simulink model "gm_hybrid_lht_vnl"  (R2019b)
settings: Solver=FixedStepDiscrete  StartTime=0.0  StopTime=inf  FixedStep=1/120e6  RelTol=1e-3
undefined symbols (not defined in the file or in its folder): bt, height, nTheta, width
libraries: hdlsllib x327, simulink x213, hdlmdlgenlib x7, dspsrcs4 x1
(part 1 of 14)
settings Model: SimulationMode=accelerator  ExtModeTrigDuration=100  Creator=rgb11127  LastModifiedBy=rgb11127
settings DataIOCC: SaveOutput=off  SaveTime=off  ReturnWorkspaceOutputs=off  StateSaveName=tmp_raccel_xout  SignalLoggingName=tmp_raccel_logsout
settings OptimizationCC: BlockReduction=off  ConditionallyExecuteInputs=off  DefaultParameterBehavior=Inlined  EfficientMapNaN2IntZero=off
settings DebuggingCC: AlgebraicLoopMsg=error  InheritedTsInSrcMsg=none  SingleTaskRateTransMsg=error  ArithmeticOperatorsInVariantConditions=warning
settings HardwareCC: ProdBitPerPointer=32  ProdBitPerSizeT=32  ProdBitPerPtrDiffT=32  ProdLargestAtomicFloat=None  ProdIntDivRoundTo=Undefined  ProdEndianess=Unspecified  ProdWordSize=32  ProdHWDeviceType=ASIC/FPGA->ASIC/FPGA  TargetBitPerPointer=64  TargetBitPerSizeT=64  TargetBitPerPtrDiffT=64  TargetLongLongMode=on  TargetIntDivRoundTo=Zero  TargetEndianess=LittleEndian  TargetWordSize=64  TargetHWDeviceType=Custom Processor->MATLAB Host Computer  ProdEqTarget=off
settings SFSimCC: CustomCodeUndefinedFunction=UseInterfaceOnly
settings RTWCC: SystemTargetFile=raccel.tlc  TemplateMakefile=raccel_default_tmf  RTWVerbose=off  RTWUseSimCustomCode=on
settings CodeAppCC: GenerateComments=off  MaxIdLength=128
settings RaccelTargetCC: GeneratePreprocessorConditionals=Use local settings  MultiInstanceERTCode=off  PreserveStateflowLocalDataDimensions=off  ExtModeMexArgs='', 0, 56287  ENABLE_SLEXEC_SSBRIDGE=1  RTWCAPIParams=on

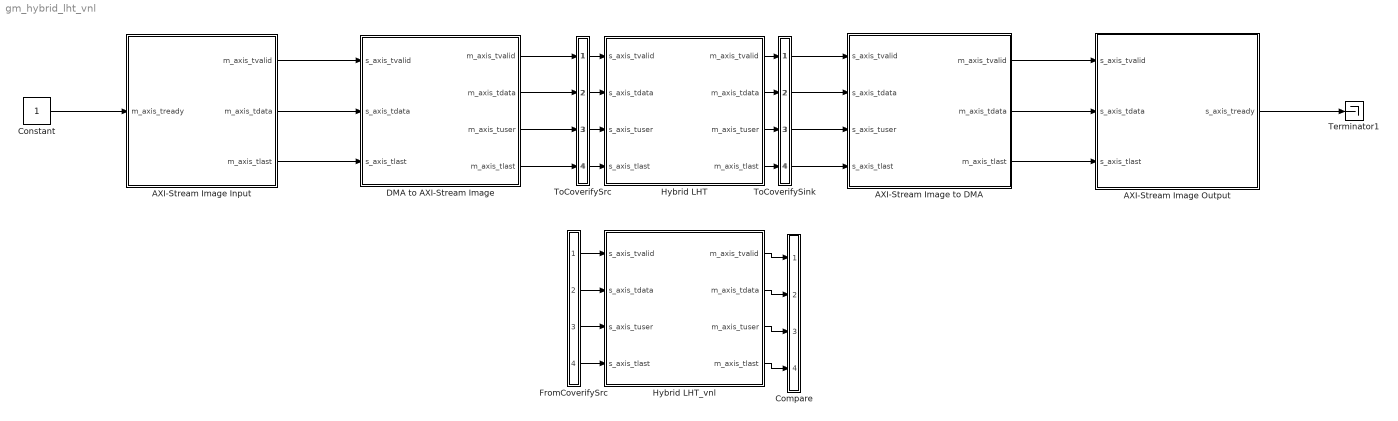
== system gm_hybrid_lht_vnl ==
  AXI-Stream Image Input : Subsystem  mask{image=bt.inputImage, clk=1/120e6}
      mask prompts: image "Input Image:"; clk "Clock Rate:"
      mask init:
      | [height, width] = size(image);
      mask DialogControl DescGroupVar Prompt: AXI-Stream Image Input
      mask DialogControl DescTextVar Prompt: This block simulates an AXI-Stream image input for interfacing to a hardware accelerator or IP Core.
      mask DialogControl ParameterGroupVar Prompt: Main
  AXI-Stream Image Output : Subsystem  mask{height=bt.nRho, width=bt.nTheta, clk=1/120e6, d=0}
      mask prompts: height "Image Height:"; width "Image Width:"; clk "Clock Rate:"; d "Frame Capture Number"
      mask DialogControl DescGroupVar Prompt: AXI-Stream Image Output
      mask DialogControl DescTextVar Prompt: Image output using the AXI-Stream interface. Simulates an AXI DMA write channel.
      mask DialogControl ParameterGroupVar Prompt: Main
  AXI-Stream Image to DMA : Subsystem  mask{height=bt.nRho, width=bt.nTheta}
      mask prompts: height "Image Height"; width "Image Width"
      mask DialogControl DescGroupVar Prompt: AXI-Stream Image to DMA
      mask DialogControl DescTextVar Prompt: Converts from the AXI-Stream video standard to AXI-Stream DMA packet.
      mask DialogControl Container2 Prompt: Main
  Compare : Subsystem
      mask Display: disp('')
  Constant : Constant  OutDataTypeStr=boolean  SampleTime=-1
  DMA to AXI-Stream Image : Subsystem  mask{height=bt.height, width=bt.width}
      mask prompts: height "Image Height:"; width "Image Width:"
      mask DialogControl DescGroupVar Prompt: DMA to AXI-Stream Image
      mask DialogControl DescTextVar Prompt: Converts an DMA AXI-Stream packet to the AXI-Stream video standard.
      mask DialogControl Container2 Prompt: Main
  FromCoverifySrc : Subsystem
      mask Display: disp('')
  Hybrid LHT : Subsystem
  Hybrid LHT_vnl : Subsystem
  Terminator1 : Terminator
  ToCoverifySink : Subsystem
      mask Display: disp('')
  ToCoverifySrc : Subsystem
      mask Display: disp('')
  wires:
  AXI-Stream Image to DMA/1(m_axis_tvalid) -> AXI-Stream Image Output/1(s_axis_tvalid)
  AXI-Stream Image to DMA/2(m_axis_tdata) -> AXI-Stream Image Output/2(s_axis_tdata)
  AXI-Stream Image to DMA/3(m_axis_tlast) -> AXI-Stream Image Output/3(s_axis_tlast)
  AXI-Stream Image Output/1(s_axis_tready) -> Terminator1/1
  AXI-Stream Image Input/3(m_axis_tlast) -> DMA to AXI-Stream Image/3(s_axis_tlast)
  AXI-Stream Image Input/2(m_axis_tdata) -> DMA to AXI-Stream Image/2(s_axis_tdata)
  AXI-Stream Image Input/1(m_axis_tvalid) -> DMA to AXI-Stream Image/1(s_axis_tvalid)
  Constant/1 -> AXI-Stream Image Input/1(m_axis_tready)
  ToCoverifySrc/1(out1) -> Hybrid LHT/1(s_axis_tvalid)
  ToCoverifySrc/2(out2) -> Hybrid LHT/2(s_axis_tdata)
  ToCoverifySrc/3(out3) -> Hybrid LHT/3(s_axis_tuser)
  ToCoverifySrc/4(out4) -> Hybrid LHT/4(s_axis_tlast)
  Hybrid LHT/1(m_axis_tvalid) -> ToCoverifySink/1(in1)
  Hybrid LHT/2(m_axis_tdata) -> ToCoverifySink/2(in2)
  Hybrid LHT/3(m_axis_tuser) -> ToCoverifySink/3(in3)
  Hybrid LHT/4(m_axis_tlast) -> ToCoverifySink/4(in4)
  DMA to AXI-Stream Image/1(m_axis_tvalid) -> ToCoverifySrc/1(in1)
  DMA to AXI-Stream Image/2(m_axis_tdata) -> ToCoverifySrc/2(in2)
  DMA to AXI-Stream Image/3(m_axis_tuser) -> ToCoverifySrc/3(in3)
  DMA to AXI-Stream Image/4(m_axis_tlast) -> ToCoverifySrc/4(in4)
  ToCoverifySink/1(out1) -> AXI-Stream Image to DMA/1(s_axis_tvalid)
  ToCoverifySink/2(out2) -> AXI-Stream Image to DMA/2(s_axis_tdata)
  ToCoverifySink/3(out3) -> AXI-Stream Image to DMA/3(s_axis_tuser)
  ToCoverifySink/4(out4) -> AXI-Stream Image to DMA/4(s_axis_tlast)
  FromCoverifySrc/1(out1) -> Hybrid LHT_vnl/1(s_axis_tvalid)
  FromCoverifySrc/2(out2) -> Hybrid LHT_vnl/2(s_axis_tdata)
  FromCoverifySrc/3(out3) -> Hybrid LHT_vnl/3(s_axis_tuser)
  FromCoverifySrc/4(out4) -> Hybrid LHT_vnl/4(s_axis_tlast)
  Hybrid LHT_vnl/1(m_axis_tvalid) -> Compare/1(in1)
  Hybrid LHT_vnl/2(m_axis_tdata) -> Compare/2(in2)
  Hybrid LHT_vnl/3(m_axis_tuser) -> Compare/3(in3)
  Hybrid LHT_vnl/4(m_axis_tlast) -> Compare/4(in4)

== system gm_hybrid_lht_vnl/AXI-Stream Image Input ==
  m_axis_tready : Inport
  Compare To Constant : simulink/Logic and Bit Operations/Compare To Constant  relop===  const=height*width-1  OutDataTypeStr=boolean
  Data Type Conversion : DataTypeConversion  OutDataTypeStr=fixdt(0, ceil(log2(max(max(double(image))))), 0)
  HDL Counter : hdlsllib/Sources/HDL Counter  CountType=Count limited  CountInit=0  CountStep=1  CountMax=width*height-1  CountFromType=Initial value  CountFrom=0  CountResetPort=off  CountLoadPort=off  CountEnbPort=on  CountDirPort=off  CountDataType=Unsigned  CountWordLen=ceil(log2(width*height))  CountFracLen=0  CountSampTime=1
      settings: SourceProductName=Simulink
  Master AXI-Stream FIFO : Subsystem  mask{depth=32}
      mask prompts: depth "FIFO Depth:"
      mask DialogControl DescGroupVar Prompt: Master AXI-Stream FIFO
      mask DialogControl DescTextVar Prompt: A custom AXI-Stream FIFO for interfacing to write channel AXI DMAs.
      mask DialogControl ParameterGroupVar Prompt: Main
  Synchronous Image Source : Subsystem
  m_axis_tvalid : Outport
  m_axis_tdata : Outport  Port=2
  m_axis_tlast : Outport  Port=3
  wires:
  Synchronous Image Source/1(Pixel) -> Data Type Conversion/1
  HDL Counter/1 -> Compare To Constant/1
  Master AXI-Stream FIFO/1(m_axis_tvalid) -> m_axis_tvalid/1
  Compare To Constant/1 -> Master AXI-Stream FIFO/3(s_axis_tlast)
  Master AXI-Stream FIFO/4(s_axis_tready) -> Synchronous Image Source/Enable, Master AXI-Stream FIFO/1(s_axis_tvalid), HDL Counter/1
  m_axis_tready/1 -> Master AXI-Stream FIFO/4(m_axis_tready)
  Master AXI-Stream FIFO/3(m_axis_tlast) -> m_axis_tlast/1
  Master AXI-Stream FIFO/2(m_axis_tdata) -> m_axis_tdata/1
  Data Type Conversion/1 -> Master AXI-Stream FIFO/2(s_axis_tdata)

== system gm_hybrid_lht_vnl/AXI-Stream Image Output ==
  s_axis_tvalid : Inport
  s_axis_tdata : Inport  Port=2
  s_axis_tlast : Inport  Port=3
  AND1 : Logic  IconShape=distinctive  AllPortsSameDT=off  OutDataTypeStr=boolean
  Compare To Constant4 : simulink/Logic and Bit Operations/Compare To Constant  relop===  const=(height)*width-1  OutDataTypeStr=boolean
  Constant : Constant  OutDataTypeStr=boolean  SampleTime=-1
  Delay2 : Delay  DelayLength=d  ShowEnablePort=on
      settings: InputPortMap=u0,e6
  Pixel to Workspace : Subsystem
  Stop Simulation1 : Stop
  Terminator : Terminator
  Total Samples Counter : hdlsllib/Sources/HDL Counter  CountType=Count limited  CountInit=0  CountStep=1  CountMax=(height)*width-1  CountFromType=Initial value  CountFrom=0  CountResetPort=off  CountLoadPort=off  CountEnbPort=on  CountDirPort=off  CountDataType=Unsigned  CountWordLen=ceil(log2((height)*width+1))  CountFracLen=0  CountSampTime=1
      settings: SourceProductName=Simulink
  s_axis_tready : Outport  VectorParamsAs1DForOutWhenUnconnected=off
  wires:
  s_axis_tdata/1 -> Pixel to Workspace/1(Pixel In)
  s_axis_tvalid/1 -> AND1/1
  AND1/1 -> Total Samples Counter/1, Pixel to Workspace/Enable
  Total Samples Counter/1 -> Compare To Constant4/1
  Compare To Constant4/1 -> Delay2/2, Delay2/1
  Delay2/1 -> Stop Simulation1/1
  s_axis_tlast/1 -> Terminator/1
  Constant/1 -> AND1/2, s_axis_tready/1

== system gm_hybrid_lht_vnl/AXI-Stream Image to DMA ==
  s_axis_tvalid : Inport
  s_axis_tdata : Inport  Port=2
  s_axis_tuser : Inport  Port=3
  s_axis_tlast : Inport  Port=4
  AND : Logic  IconShape=distinctive  AllPortsSameDT=off  OutDataTypeStr=boolean
  Compare To Constant : simulink/Logic and Bit Operations/Compare To Constant  relop===  const=height*width-1  OutDataTypeStr=boolean
  Data Type Conversion : DataTypeConversion  OutDataTypeStr=uint32
  Output Counter : hdlsllib/Sources/HDL Counter  CountType=Count limited  CountInit=0  CountStep=1  CountMax=height*width-1  CountFromType=Initial value  CountFrom=0  CountResetPort=off  CountLoadPort=off  CountEnbPort=on  CountDirPort=off  CountDataType=Unsigned  CountWordLen=ceil(log2(height*width))  CountFracLen=0  CountSampTime=1
      settings: SourceProductName=Simulink
  Terminator : Terminator
  Terminator1 : Terminator
  m_axis_tvalid : Outport
  m_axis_tdata : Outport  Port=2
  m_axis_tlast : Outport  Port=3
  wires:
  AND/1 -> m_axis_tlast/1
  Compare To Constant/1 -> AND/1
  Output Counter/1 -> Compare To Constant/1
  s_axis_tuser/1 -> Terminator1/1
  s_axis_tlast/1 -> Terminator/1
  s_axis_tvalid/1 -> Output Counter/1, m_axis_tvalid/1, AND/2
  s_axis_tdata/1 -> Data Type Conversion/1
  Data Type Conversion/1 -> m_axis_tdata/1

== system gm_hybrid_lht_vnl/Compare ==
  in1 : Inport
  in2 : Inport  Port=2
  in3 : Inport  Port=3
  in4 : Inport  Port=4
  Assert_m_axis_tdata : Subsystem
  Assert_m_axis_tlast : Subsystem
  Assert_m_axis_tuser : Subsystem
  Assert_m_axis_tvalid : Subsystem
  CleanupScopes : Subsystem
      settings: OpenFcn=|
      | blkName = gcb; %self block
      | idx = regexp(blkName, '/CleanupScopes$', 'once');
      | blkParent = blkName(1:idx-1);
      | blks=find_system(blkParent, 'LookUnderMasks', 'all','blocktype', 'Scope');
      | for itr = 1:length(blks)
      | 	 hScopeCfg = get_param(blks{itr},'ScopeConfiguration');
      | 	 hScopeCfg.Visible = ~ hScopeCfg.Visible;
      | end
      | drawnow;
      mask Display: fprintf(message('hdlcoder:cosim:vnl_dblclick').getString());
  Enable : Subsystem
      settings: OpenFcn=|
      | blkName = gcb;
      | idx = regexp(blkName, '/Enable$', 'once');
      | blkParent = blkName(1:idx-1);
      | blks=find_system(blkParent, 'LookUnderMasks', 'all','blocktype', 'Assertion');
      | e = get_param(blks{1}, 'Enabled');
      | if strcmp(e, 'on'), f= 'off';, else, f = 'on';, end
      | for ii=1:length(blks), set_param(blks{ii}, 'Enabled', f);, end
      | set_param(gcb, 'MaskDisplay',['fprintf(message(''hdlcoder:cosim:vnl_dblclick_assertions'',','''',upper(e),'''',').getString())']);
      mask Display: fprintf(message('hdlcoder:cosim:vnl_dblclick_assertions','OFF').getString());
  pathdelay{1..4} (4 alike) : Delay
  wires:
  in1/1 -> pathdelay1/1
  pathdelay1/1 -> Assert_m_axis_tvalid/1(cosim)
  [out1] -> Assert_m_axis_tvalid/2(dut)
  in2/1 -> pathdelay2/1
  pathdelay2/1 -> Assert_m_axis_tdata/1(cosim)
  [out2] -> Assert_m_axis_tdata/2(dut)
  in3/1 -> pathdelay3/1
  pathdelay3/1 -> Assert_m_axis_tuser/1(cosim)
  [out3] -> Assert_m_axis_tuser/2(dut)
  in4/1 -> pathdelay4/1
  pathdelay4/1 -> Assert_m_axis_tlast/1(cosim)
  [out4] -> Assert_m_axis_tlast/2(dut)

== system gm_hybrid_lht_vnl/DMA to AXI-Stream Image ==
  s_axis_tvalid : Inport
  s_axis_tdata : Inport  Port=2
  s_axis_tlast : Inport  Port=3
  AND : Logic  IconShape=distinctive  AllPortsSameDT=off  OutDataTypeStr=boolean
  AND1 : Logic  IconShape=distinctive  AllPortsSameDT=off  OutDataTypeStr=boolean
  AND2 : Logic  IconShape=distinctive  AllPortsSameDT=off  OutDataTypeStr=boolean
  Compare To Constant : simulink/Logic and Bit Operations/Compare To Constant  relop===  const=width-1  OutDataTypeStr=boolean
  Compare To Zero : simulink/Logic and Bit Operations/Compare To Zero  relop===  OutDataTypeStr=boolean
  Compare To Zero1 : simulink/Logic and Bit Operations/Compare To Zero  relop===  OutDataTypeStr=boolean
  Terminator : Terminator
  X Counter : hdlsllib/Sources/HDL Counter  CountType=Count limited  CountInit=0  CountStep=1  CountMax=width-1  CountFromType=Initial value  CountFrom=0  CountResetPort=off  CountLoadPort=off  CountEnbPort=on  CountDirPort=off  CountDataType=Unsigned  CountWordLen=ceil(log2(width))  CountFracLen=0  CountSampTime=1
      settings: SourceProductName=Simulink
  Y Counter : hdlsllib/Sources/HDL Counter  CountType=Count limited  CountInit=0  CountStep=1  CountMax=height-1  CountFromType=Initial value  CountFrom=0  CountResetPort=off  CountLoadPort=off  CountEnbPort=on  CountDirPort=off  CountDataType=Unsigned  CountWordLen=ceil(log2(height))  CountFracLen=0  CountSampTime=1
      settings: SourceProductName=Simulink
  m_axis_tvalid : Outport
  m_axis_tdata : Outport  Port=2
  m_axis_tuser : Outport  Port=3
  m_axis_tlast : Outport  Port=4
  wires:
  s_axis_tdata/1 -> m_axis_tdata/1
  s_axis_tvalid/1 -> X Counter/1, AND2/1, AND1/1, m_axis_tvalid/1
  X Counter/1 -> Compare To Zero1/1, Compare To Constant/1
  Y Counter/1 -> Compare To Zero/1
  Compare To Zero1/1 -> AND/1
  Compare To Zero/1 -> AND/2
  s_axis_tlast/1 -> Terminator/1
  AND/1 -> AND1/2
  AND1/1 -> m_axis_tuser/1
  Compare To Constant/1 -> AND2/2, Y Counter/1
  AND2/1 -> m_axis_tlast/1

== system gm_hybrid_lht_vnl/FromCoverifySrc ==
  out1 : Outport
  out2 : Outport  Port=2
  out3 : Outport  Port=3
  out4 : Outport  Port=4
  wires:
  [in1] -> out1/1
  [in2] -> out2/1
  [in3] -> out3/1
  [in4] -> out4/1

== system gm_hybrid_lht_vnl/Hybrid LHT ==
  s_axis_tvalid : Inport  OutDataTypeStr=boolean  PortDimensions=1  SampleTime=8.33333333333333e-09
  s_axis_tdata : Inport  Port=2  OutDataTypeStr=fixdt(0, 9, 0)  PortDimensions=1  SampleTime=8.33333333333333e-09
  s_axis_tuser : Inport  Port=3  OutDataTypeStr=boolean  PortDimensions=1  SampleTime=8.33333333333333e-09
  s_axis_tlast : Inport  Port=4  OutDataTypeStr=boolean  PortDimensions=1  SampleTime=8.33333333333333e-09
  Hybrid LHT Accumulator : Subsystem  mask{height=double(480), width=double(640), theta=reshape(double([0 1 2 3 4 5 6 7 8 9 10 11 12 13 14 15 16 17 18 19 20 21 22 23 24 25 26 27 28 29 30 31 32 33 34 35 36 37 38 39 40 41 42 43 44 45 46 47 48 49 50 51 52 53 54 55 56 57 58 59 60 61 62 63 64 65 66 67 68 69 70 71 72 73 74 75 76 77 78 79 80 81 82 83 84 85 86 87 88 89 90 91 92 93 94 95 96 97 98 99 100 101 102 103 104 105 106 107 108 109 110 111 112 113 114 115 116 117 118 119 120 121 122 123 124 125 126 127 128 129 130 131 132 133 134 135 136 137 138 139 140 141 142 143 144 145 146 147 148 149 150 151 152 153 154 155 156 157 158 159 160 161 162 163 164 165 166 167 168 169 170 171 172 173 174 175 176 177 178 179]).', [1  180])}
      mask prompts: height "Image Height:"; width "Image Width:"; theta "Orientations:"
      mask init:
      | maxRho = ceil(sqrt((height/2)^2+(width/2)^2));
      | nRho = maxRho*2;
      | [~, nTheta] = size(theta);
      | 
      | voteWL = ceil(log2(2*maxRho));
  Hybrid LHT Kernel : Subsystem  mask{height=double(480), width=double(640), theta=reshape(double([0 1 2 3 4 5 6 7 8 9 10 11 12 13 14 15 16 17 18 19 20 21 22 23 24 25 26 27 28 29 30 31 32 33 34 35 36 37 38 39 40 41 42 43 44 45 46 47 48 49 50 51 52 53 54 55 56 57 58 59 60 61 62 63 64 65 66 67 68 69 70 71 72 73 74 75 76 77 78 79 80 81 82 83 84 85 86 87 88 89 90 91 92 93 94 95 96 97 98 99 100 101 102 103 104 105 106 107 108 109 110 111 112 113 114 115 116 117 118 119 120 121 122 123 124 125 126 127 128 129 130 131 132 133 134 135 136 137 138 139 140 141 142 143 144 145 146 147 148 149 150 151 152 153 154 155 156 157 158 159 160 161 162 163 164 165 166 167 168 169 170 171 172 173 174 175 176 177 178 179]).', [1  180])}
      mask prompts: height "Image Height:"; width "Image Width:"; theta "Orientations:"
      mask init:
      | % Get number of orientations to operate across
      | [~, nTheta] = size(theta);
      | 
      | % Get discretisation step of theta
      | if nTheta > 1
      |     dTheta = theta(end) - theta(end-1);
      | else
      |     dTheta = 1;
      | end
      | 
      | % Get the maximum magnitude of displacement
      | maxRho = ceil(sqrt((height/2)^2+(width/2)^2));
      | 
      | % Get the number of bits required to vote correctly
      | voteWL = ceil(log2(maxRho*2));
      | 
      | % Get the number of division possible
      | if nTheta < floor(36/voteWL)
      |     L = nTheta;
      | else
      |     L = floor(36/voteWL);
      | end
      | 
      | % Set lambda, the number of orientations to operate across per gradient
      | % orientation given
      | lambda = floor(nTheta/(2*L));
      | 
      | % Determine if the number of orientations is odd. This will prevent over
      | % use of the parameter space.
      | if lambda == 0
      |     subflag = 0;
      | else
      |     subflag = ~mod(nTheta/(L), 2);
      | end
      | 
      | % Get the limits so that we can determine the number of bits to shift
      | % the votes
      | U = floor(nTheta/L):floor(nTheta/L):nTheta;
      | D = 0:floor(nTheta/L):nTheta-1;
  delayMatch : Delay  DelayLength=double(2)  InitialCondition=0  SampleTime=8.33333333333333e-09
  delayMatch1 : Delay  DelayLength=double(2)  InitialCondition=0  SampleTime=8.33333333333333e-09
  m_axis_tvalid : Outport
  m_axis_tdata : Outport  Port=2
  m_axis_tuser : Outport  Port=3
  m_axis_tlast : Outport  Port=4
  wires:
  Hybrid LHT Accumulator/4(m_axis_tlast) -> delayMatch1/1
  Hybrid LHT Accumulator/1(m_axis_tvalid) -> delayMatch/1
  Hybrid LHT Kernel/6(shift) -> Hybrid LHT Accumulator/6(shift)
  Hybrid LHT Kernel/5(edge) -> Hybrid LHT Accumulator/5(edge)
  Hybrid LHT Kernel/4(hough_param) -> Hybrid LHT Accumulator/4(hough_param)
  Hybrid LHT Kernel/3(m_axis_tlast) -> Hybrid LHT Accumulator/3(s_axis_tlast)
  Hybrid LHT Kernel/2(m_axis_tuser) -> Hybrid LHT Accumulator/2(s_axis_tuser)
  Hybrid LHT Kernel/1(m_axis_tvalid) -> Hybrid LHT Accumulator/1(s_axis_tvalid)
  delayMatch1/1 -> m_axis_tlast/1
  Hybrid LHT Accumulator/3(m_axis_tuser) -> m_axis_tuser/1
  Hybrid LHT Accumulator/2(m_axis_tdata) -> m_axis_tdata/1
  delayMatch/1 -> m_axis_tvalid/1
  s_axis_tlast/1 -> Hybrid LHT Kernel/4(s_axis_tlast)
  s_axis_tuser/1 -> Hybrid LHT Kernel/3(s_axis_tuser)
  s_axis_tdata/1 -> Hybrid LHT Kernel/2(s_axis_tdata)
  s_axis_tvalid/1 -> Hybrid LHT Kernel/1(s_axis_tvalid)

== system gm_hybrid_lht_vnl/Hybrid LHT_vnl ==
  s_axis_tvalid : Inport
  s_axis_tdata : Inport  Port=2
  s_axis_tuser : Inport  Port=3
  s_axis_tlast : Inport  Port=4
  Hybrid LHT Accumulator : Subsystem  mask{height=bt.height, width=bt.width, theta=bt.theta}
      mask prompts: height "Image Height:"; width "Image Width:"; theta "Orientations:"
      mask init:
      | maxRho = ceil(sqrt((height/2)^2+(width/2)^2));
      | nRho = maxRho*2;
      | [~, nTheta] = size(theta);
      | 
      | voteWL = ceil(log2(2*maxRho));
      mask DialogControl ParameterGroupVar Prompt: Main
  Hybrid LHT Kernel : Subsystem  mask{height=bt.height, width=bt.width, theta=bt.theta}
      mask prompts: height "Image Height:"; width "Image Width:"; theta "Orientations:"
      mask init: same as gm_hybrid_lht_vnl/Hybrid LHT/Hybrid LHT Kernel
      mask DialogControl ParameterGroupVar Prompt: Main
  m_axis_tvalid : Outport
  m_axis_tdata : Outport  Port=2
  m_axis_tuser : Outport  Port=3
  m_axis_tlast : Outport  Port=4
  wires:
  Hybrid LHT Kernel/1(m_axis_tvalid) -> Hybrid LHT Accumulator/1(s_axis_tvalid)
  Hybrid LHT Kernel/2(m_axis_tuser) -> Hybrid LHT Accumulator/2(s_axis_tuser)
  Hybrid LHT Kernel/3(m_axis_tlast) -> Hybrid LHT Accumulator/3(s_axis_tlast)
  Hybrid LHT Kernel/4(hough_param) -> Hybrid LHT Accumulator/4(hough_param)
  Hybrid LHT Kernel/5(edge) -> Hybrid LHT Accumulator/5(edge)
  Hybrid LHT Kernel/6(shift) -> Hybrid LHT Accumulator/6(shift)
  Hybrid LHT Accumulator/1(m_axis_tvalid) -> m_axis_tvalid/1
  Hybrid LHT Accumulator/2(m_axis_tdata) -> m_axis_tdata/1
  Hybrid LHT Accumulator/3(m_axis_tuser) -> m_axis_tuser/1
  Hybrid LHT Accumulator/4(m_axis_tlast) -> m_axis_tlast/1
  s_axis_tvalid/1 -> Hybrid LHT Kernel/1(s_axis_tvalid)
  s_axis_tdata/1 -> Hybrid LHT Kernel/2(s_axis_tdata)
  s_axis_tuser/1 -> Hybrid LHT Kernel/3(s_axis_tuser)
  s_axis_tlast/1 -> Hybrid LHT Kernel/4(s_axis_tlast)

== system gm_hybrid_lht_vnl/ToCoverifySink ==
  in1 : Inport
  in2 : Inport  Port=2
  in3 : Inport  Port=3
  in4 : Inport  Port=4
  out1 : Outport
  out2 : Outport  Port=2
  out3 : Outport  Port=3
  out4 : Outport  Port=4
  tag scope: out1=global, out2=global, out3=global, out4=global
  wires:
  in1/1 -> out1/1, [out1]
  in2/1 -> out2/1, [out2]
  in3/1 -> out3/1, [out3]
  in4/1 -> out4/1, [out4]

== system gm_hybrid_lht_vnl/ToCoverifySrc ==
  in1 : Inport
  in2 : Inport  Port=2
  in3 : Inport  Port=3
  in4 : Inport  Port=4
  out1 : Outport
  out2 : Outport  Port=2
  out3 : Outport  Port=3
  out4 : Outport  Port=4
  tag scope: in1=global, in2=global, in3=global, in4=global
  wires:
  in1/1 -> out1/1, [in1]
  in2/1 -> out2/1, [in2]
  in3/1 -> out3/1, [in3]
  in4/1 -> out4/1, [in4]

== system gm_hybrid_lht_vnl/AXI-Stream Image Input/Master AXI-Stream FIFO ==
  s_axis_tvalid : Inport
  s_axis_tdata : Inport  Port=2
  s_axis_tlast : Inport  Port=3
  m_axis_tready : Inport  Port=4
  AND : Logic  IconShape=distinctive  AllPortsSameDT=off  OutDataTypeStr=boolean
  "Compare To Constant " : simulink/Logic and Bit Operations/Compare To Constant  relop=>=  const=floor(depth/2)  OutDataTypeStr=boolean
  Delay : Delay  DelayLength=1
  HDL FIFO TDATA : hdlsllib/HDL RAMs/HDL FIFO  fifo_size=depth  mode=Classic  ratio=1  push_msg=Error  pop_msg=Error  show_empty=on  show_full=off  show_num=on  LabelModeActiveChoice_Mode=Classic
      settings: SourceProductName=Simulink  SourceProductBaseCode=SL
  HDL FIFO TLAST : hdlsllib/HDL RAMs/HDL FIFO  fifo_size=depth  mode=Classic  ratio=1  push_msg=Error  pop_msg=Error  show_empty=off  show_full=off  show_num=off  LabelModeActiveChoice_Mode=Classic
      settings: SourceProductName=Simulink  SourceProductBaseCode=SL
  NOT : Logic  Operator=NOT  IconShape=distinctive  AllPortsSameDT=off  OutDataTypeStr=boolean
  NOT1 : Logic  Operator=NOT  IconShape=distinctive  AllPortsSameDT=off  OutDataTypeStr=boolean
  m_axis_tvalid : Outport  VectorParamsAs1DForOutWhenUnconnected=off
  m_axis_tdata : Outport  Port=2  VectorParamsAs1DForOutWhenUnconnected=off
  m_axis_tlast : Outport  Port=3  VectorParamsAs1DForOutWhenUnconnected=off
  s_axis_tready : Outport  Port=4
  wires:
  HDL FIFO TDATA/1 -> m_axis_tdata/1
  HDL FIFO TLAST/1 -> m_axis_tlast/1
  HDL FIFO TDATA/2 -> NOT/1
  AND/1 -> HDL FIFO TLAST/3, HDL FIFO TDATA/3
  NOT/1 -> Delay/1, AND/2
  m_axis_tready/1 -> AND/1
  HDL FIFO TDATA/3 -> "Compare To Constant "/1
  NOT1/1 -> s_axis_tready/1
  "Compare To Constant "/1 -> NOT1/1
  s_axis_tlast/1 -> HDL FIFO TLAST/1
  s_axis_tdata/1 -> HDL FIFO TDATA/1
  s_axis_tvalid/1 -> HDL FIFO TLAST/2, HDL FIFO TDATA/2
  Delay/1 -> m_axis_tvalid/1

== system gm_hybrid_lht_vnl/AXI-Stream Image Input/Synchronous Image Source ==
  Enable : EnablePort
  Signal From Workspace : dspsrcs4/Signal From Workspace  X=reshape((double(image))', [height*width, 1])  Ts=clk  nsamps=1  OutputAfterFinalValue=Cyclic repetition  ignoreOrWarnInputAndFrameLengths=off  OutputFrames=off
  Pixel : Outport
  wires:
  Signal From Workspace/1 -> Pixel/1

== system gm_hybrid_lht_vnl/AXI-Stream Image Output/Pixel to Workspace ==
  Pixel In : Inport
  Enable : EnablePort
  To Workspace : ToWorkspace  VariableName=simout  SampleTime=-1
      settings: MaxDataPoints=height*width  Save2DSignal=2-D array (concatenate along first dimension)
  wires:
  Pixel In/1 -> To Workspace/1

== system gm_hybrid_lht_vnl/Compare/Assert_m_axis_tdata ==
  cosim : Inport
  dut : Inport  Port=2
  AssertEq : Assertion  StopWhenAssertionFail=off
  Compare To Zero : simulink/Logic and Bit Operations/Compare To Zero  relop===  OutDataTypeStr=boolean
  Constant1 : Constant  Value=0  OutDataTypeStr=Inherit: Inherit via back propagation  SampleTime=-1
  Counter : simulink/Sources/Counter Free-Running  NumBits=32  tsamp=-1
  IgnoreCycles : Constant  Value=2  OutDataTypeStr=Inherit: Inherit via back propagation  SampleTime=-1
  Relational Operator : RelationalOperator  Operator=<  OutDataTypeStr=boolean  RndMeth=Nearest
  Relational Operator1 : RelationalOperator  Operator===  OutDataTypeStr=boolean  RndMeth=Nearest
  Switch : Switch  Criteria=u2 ~= 0
  Switch1 : Switch  Criteria=u2 ~= 0
  compare: m_axis_tdata : Scope  NumInputPorts=3
  wires:
  Compare To Zero/1 -> compare: m_axis_tdata/3
  Relational Operator1/1 -> Compare To Zero/1, AssertEq/1  "err"
  Switch1/1 -> compare: m_axis_tdata/1, Relational Operator1/1
  Switch/1 -> compare: m_axis_tdata/2, Relational Operator1/2
  Constant1/1 -> Switch/1, Switch1/1
  Relational Operator/1 -> Switch/2, Switch1/2
  cosim/1 -> Switch1/3  "cosim"
  dut/1 -> Switch/3  "dut ref"
  Counter/1 -> Relational Operator/1
  IgnoreCycles/1 -> Relational Operator/2

== system gm_hybrid_lht_vnl/Compare/Assert_m_axis_tlast ==
  cosim : Inport
  dut : Inport  Port=2
  AssertEq : Assertion  StopWhenAssertionFail=off
  Compare To Zero : simulink/Logic and Bit Operations/Compare To Zero  relop===  OutDataTypeStr=boolean
  Constant1 : Constant  Value=0  OutDataTypeStr=Inherit: Inherit via back propagation  SampleTime=-1
  Counter : simulink/Sources/Counter Free-Running  NumBits=32  tsamp=-1
  IgnoreCycles : Constant  Value=2  OutDataTypeStr=Inherit: Inherit via back propagation  SampleTime=-1
  Relational Operator : RelationalOperator  Operator=<  OutDataTypeStr=boolean  RndMeth=Nearest
  Relational Operator1 : RelationalOperator  Operator===  OutDataTypeStr=boolean  RndMeth=Nearest
  Switch : Switch  Criteria=u2 ~= 0
  Switch1 : Switch  Criteria=u2 ~= 0
  compare: m_axis_tlast : Scope  NumInputPorts=3
  wires:
  Compare To Zero/1 -> compare: m_axis_tlast/3
  Relational Operator1/1 -> Compare To Zero/1, AssertEq/1  "err"
  Switch1/1 -> compare: m_axis_tlast/1, Relational Operator1/1
  Switch/1 -> compare: m_axis_tlast/2, Relational Operator1/2
  Constant1/1 -> Switch/1, Switch1/1
  Relational Operator/1 -> Switch/2, Switch1/2
  cosim/1 -> Switch1/3  "cosim"
  dut/1 -> Switch/3  "dut ref"
  Counter/1 -> Relational Operator/1
  IgnoreCycles/1 -> Relational Operator/2

== system gm_hybrid_lht_vnl/Compare/Assert_m_axis_tuser ==
  cosim : Inport
  dut : Inport  Port=2
  AssertEq : Assertion  StopWhenAssertionFail=off
  Compare To Zero : simulink/Logic and Bit Operations/Compare To Zero  relop===  OutDataTypeStr=boolean
  Constant1 : Constant  Value=0  OutDataTypeStr=Inherit: Inherit via back propagation  SampleTime=-1
  Counter : simulink/Sources/Counter Free-Running  NumBits=32  tsamp=-1
  IgnoreCycles : Constant  Value=2  OutDataTypeStr=Inherit: Inherit via back propagation  SampleTime=-1
  Relational Operator : RelationalOperator  Operator=<  OutDataTypeStr=boolean  RndMeth=Nearest
  Relational Operator1 : RelationalOperator  Operator===  OutDataTypeStr=boolean  RndMeth=Nearest
  Switch : Switch  Criteria=u2 ~= 0
  Switch1 : Switch  Criteria=u2 ~= 0
  compare: m_axis_tuser : Scope  NumInputPorts=3
  wires:
  Compare To Zero/1 -> compare: m_axis_tuser/3
  Relational Operator1/1 -> Compare To Zero/1, AssertEq/1  "err"
  Switch1/1 -> compare: m_axis_tuser/1, Relational Operator1/1
  Switch/1 -> compare: m_axis_tuser/2, Relational Operator1/2
  Constant1/1 -> Switch/1, Switch1/1
  Relational Operator/1 -> Switch/2, Switch1/2
  cosim/1 -> Switch1/3  "cosim"
  dut/1 -> Switch/3  "dut ref"
  Counter/1 -> Relational Operator/1
  IgnoreCycles/1 -> Relational Operator/2

== system gm_hybrid_lht_vnl/Compare/Assert_m_axis_tvalid ==
  cosim : Inport
  dut : Inport  Port=2
  AssertEq : Assertion  StopWhenAssertionFail=off
  Compare To Zero : simulink/Logic and Bit Operations/Compare To Zero  relop===  OutDataTypeStr=boolean
  Constant1 : Constant  Value=0  OutDataTypeStr=Inherit: Inherit via back propagation  SampleTime=-1
  Counter : simulink/Sources/Counter Free-Running  NumBits=32  tsamp=-1
  IgnoreCycles : Constant  Value=2  OutDataTypeStr=Inherit: Inherit via back propagation  SampleTime=-1
  Relational Operator : RelationalOperator  Operator=<  OutDataTypeStr=boolean  RndMeth=Nearest
  Relational Operator1 : RelationalOperator  Operator===  OutDataTypeStr=boolean  RndMeth=Nearest
  Switch : Switch  Criteria=u2 ~= 0
  Switch1 : Switch  Criteria=u2 ~= 0
  compare: m_axis_tvalid : Scope  NumInputPorts=3
  wires:
  Compare To Zero/1 -> compare: m_axis_tvalid/3
  Relational Operator1/1 -> Compare To Zero/1, AssertEq/1  "err"
  Switch1/1 -> compare: m_axis_tvalid/1, Relational Operator1/1
  Switch/1 -> compare: m_axis_tvalid/2, Relational Operator1/2
  Constant1/1 -> Switch/1, Switch1/1
  Relational Operator/1 -> Switch/2, Switch1/2
  cosim/1 -> Switch1/3  "cosim"
  dut/1 -> Switch/3  "dut ref"
  Counter/1 -> Relational Operator/1
  IgnoreCycles/1 -> Relational Operator/2

== system gm_hybrid_lht_vnl/Compare/CleanupScopes ==

== system gm_hybrid_lht_vnl/Compare/Enable ==

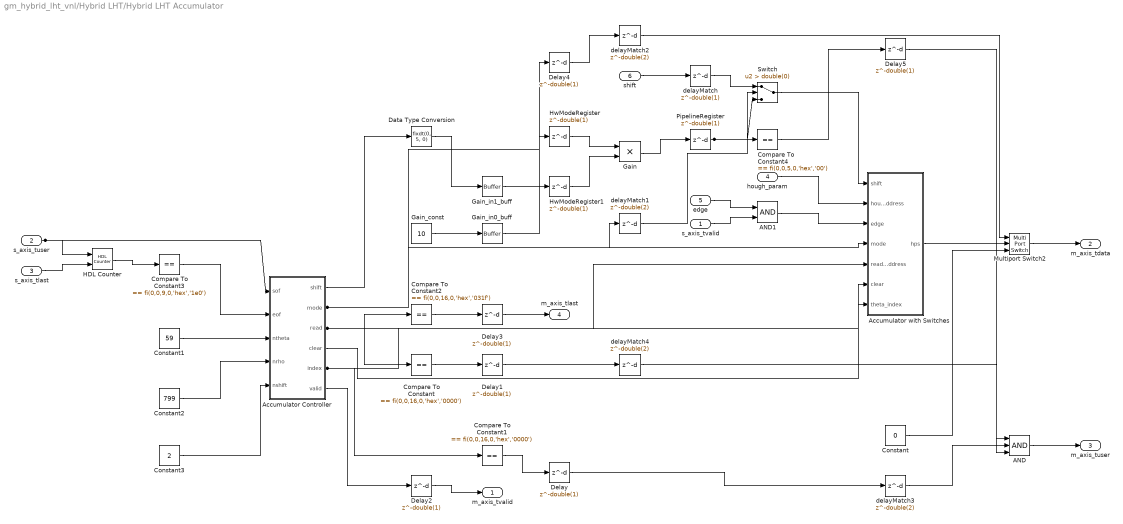
== system gm_hybrid_lht_vnl/Hybrid LHT/Hybrid LHT Accumulator ==
  s_axis_tvalid : Inport  OutDataTypeStr=boolean  PortDimensions=1  SampleTime=8.33333333333333e-09
  s_axis_tuser : Inport  Port=2  OutDataTypeStr=boolean  PortDimensions=1  SampleTime=8.33333333333333e-09
  s_axis_tlast : Inport  Port=3  OutDataTypeStr=boolean  PortDimensions=1  SampleTime=8.33333333333333e-09
  hough_param : Inport  Port=4  OutDataTypeStr=fixdt(0, 10, 0)  PortDimensions=[1 60]  SampleTime=8.33333333333333e-09
  edge : Inport  Port=5  OutDataTypeStr=fixdt(0, 1, 0)  PortDimensions=1  SampleTime=8.33333333333333e-09
  shift : Inport  Port=6  OutDataTypeStr=fixdt(0, 6, 0)  PortDimensions=[1 60]  SampleTime=8.33333333333333e-09
  AND : Logic  Inputs=3  AllPortsSameDT=off  OutDataTypeStr=boolean  SampleTime=8.33333333333333e-09
  AND1 : Logic  AllPortsSameDT=off  OutDataTypeStr=boolean  SampleTime=8.33333333333333e-09
  Accumulator Controller : Subsystem
  Accumulator with Switches : Subsystem
  Compare To Constant : simulink/Logic and Bit Operations/Compare To Constant  relop===  const=fi(0,0,16,0,'hex','0000')  OutDataTypeStr=boolean
  Compare To Constant1 : simulink/Logic and Bit Operations/Compare To Constant  relop===  const=fi(0,0,16,0,'hex','0000')  OutDataTypeStr=boolean
  Compare To Constant2 : simulink/Logic and Bit Operations/Compare To Constant  relop===  const=fi(0,0,16,0,'hex','031f')  OutDataTypeStr=boolean
  Compare To Constant3 : simulink/Logic and Bit Operations/Compare To Constant  relop===  const=fi(0,0,9,0,'hex','1e0')  OutDataTypeStr=boolean
  Compare To Constant4 : simulink/Logic and Bit Operations/Compare To Constant  relop===  const=fi(0,0,5,0,'hex','00')  OutDataTypeStr=boolean
  Constant : Constant  Value=0  OutDataTypeStr=fixdt(0, 10, 0)  SampleTime=-1
  Constant1 : Constant  Value=59  OutDataTypeStr=uint16  SampleTime=-1
  Constant2 : Constant  Value=799  OutDataTypeStr=uint16  SampleTime=-1
  Constant3 : Constant  Value=2  OutDataTypeStr=fixdt(0, 3, 0)  SampleTime=-1
  Data Type Conversion : DataTypeConversion  OutDataTypeStr=fixdt(0, 5, 0)  SampleTime=8.33333333333333e-09
  Delay{,1..5} (6 alike) : Delay  DelayLength=double(1)  InitialCondition=0  SampleTime=8.33333333333333e-09
  Gain : Product  Inputs=**  OutDataTypeStr=fixdt(0, 5, 0)  SampleTime=8.33333333333333e-09
  Gain_const : Constant  Value=10  OutDataTypeStr=fixdt(0, 5, 1)  SampleTime=-1
  Gain_in0_buff : hdlmdlgenlib/Buffer
      settings: SourceProductName=Simulink  SourceProductBaseCode=SL
  Gain_in1_buff : hdlmdlgenlib/Buffer
      settings: SourceProductName=Simulink  SourceProductBaseCode=SL
  HDL Counter : hdlsllib/Sources/HDL Counter  CountType=Count limited  CountInit=double(0)  CountStep=double(1)  CountMax=double(480)  CountFromType=Initial value  CountFrom=double(0)  CountResetPort=on  CountLoadPort=off  CountEnbPort=on  CountDirPort=off  CountDataType=Unsigned  CountWordLen=9  CountFracLen=0  CountSampTime=8.33333333333333e-09
      settings: SourceProductName=Simulink
  HwModeRegister : Delay  DelayLength=double(1)  InitialCondition=0  SampleTime=8.33333333333333e-09
  HwModeRegister1 : Delay  DelayLength=double(1)  InitialCondition=0  SampleTime=8.33333333333333e-09
  Multiport Switch2 : MultiPortSwitch  DataPortOrder=Zero-based contiguous  Inputs=2  DiagnosticForDefault=None  zeroidx=on  OutDataTypeStr=fixdt(0, 10, 0)  SampleTime=8.33333333333333e-09
  PipelineRegister : Delay  DelayLength=double(1)  InitialCondition=0  SampleTime=8.33333333333333e-09
  Switch : Switch  Criteria=u2 > Threshold  Threshold=double(0)  OutDataTypeStr=fixdt(0, 6, 0)  SampleTime=8.33333333333333e-09
  delayMatch : Delay  DelayLength=double(1)  InitialCondition=0  SampleTime=8.33333333333333e-09
  delayMatch{1..4} (4 alike) : Delay  DelayLength=double(2)  InitialCondition=0  SampleTime=8.33333333333333e-09
  m_axis_tvalid : Outport
  m_axis_tdata : Outport  Port=2
  m_axis_tuser : Outport  Port=3
  m_axis_tlast : Outport  Port=4
  wires:
  Gain_in1_buff/1 -> HwModeRegister1/1
  Gain_in0_buff/1 -> HwModeRegister/1
  HwModeRegister1/1 -> Gain/2
  HwModeRegister/1 -> Gain/1
  Gain/1 -> PipelineRegister/1
  Delay1/1 -> delayMatch4/1
  Delay/1 -> delayMatch3/1
  Delay4/1 -> delayMatch2/1
  Accumulator Controller/2(mode) -> Accumulator with Switches/4(mode), Delay4/1, delayMatch1/1
  shift/1 -> delayMatch/1
  edge/1 -> AND1/1
  hough_param/1 -> Accumulator with Switches/2(hough_address)
  s_axis_tlast/1 -> HDL Counter/2
  s_axis_tuser/1 -> Accumulator Controller/1(sof), HDL Counter/1
  s_axis_tvalid/1 -> AND1/2
  Gain_const/1 -> Gain_in0_buff/1
  Switch/1 -> Accumulator with Switches/1(shift)
  Multiport Switch2/1 -> m_axis_tdata/1
  HDL Counter/1 -> Compare To Constant3/1
  PipelineRegister/1 -> Compare To Constant4/1, Switch/3
  Delay5/1 -> AND/1
  delayMatch2/1 -> Multiport Switch2/1
  Delay3/1 -> m_axis_tlast/1
  Delay2/1 -> m_axis_tvalid/1
  delayMatch4/1 -> AND/3
  delayMatch3/1 -> AND/2
  Data Type Conversion/1 -> Gain_in1_buff/1
  Constant3/1 -> Accumulator Controller/5(nshift)
  Constant2/1 -> Accumulator Controller/4(nrho)
  Constant1/1 -> Accumulator Controller/3(ntheta)
  Constant/1 -> Multiport Switch2/3
  Compare To Constant4/1 -> Delay5/1
  Compare To Constant3/1 -> Accumulator Controller/2(eof)
  Compare To Constant2/1 -> Delay3/1
  Compare To Constant1/1 -> Delay/1
  Compare To Constant/1 -> Delay1/1
  Accumulator with Switches/1(hps) -> Multiport Switch2/2
  Accumulator Controller/6(valid) -> Delay2/1
  Accumulator Controller/5(index) -> Accumulator with Switches/7(theta_index), Compare To Constant1/1
  Accumulator Controller/4(clear) -> Accumulator with Switches/6(clear)
  Accumulator Controller/3(read) -> Accumulator with Switches/5(read_address), Compare To Constant/1, Compare To Constant2/1
  delayMatch1/1 -> Switch/2
  Accumulator Controller/1(shift) -> Data Type Conversion/1
  AND1/1 -> Accumulator with Switches/3(edge)
  AND/1 -> m_axis_tuser/1
  delayMatch/1 -> Switch/1

== system gm_hybrid_lht_vnl/Hybrid LHT/Hybrid LHT Kernel ==
  s_axis_tvalid : Inport  OutDataTypeStr=boolean  PortDimensions=1  SampleTime=8.33333333333333e-09
  s_axis_tdata : Inport  Port=2  OutDataTypeStr=fixdt(0, 9, 0)  PortDimensions=1  SampleTime=8.33333333333333e-09
  s_axis_tuser : Inport  Port=3  OutDataTypeStr=boolean  PortDimensions=1  SampleTime=8.33333333333333e-09
  s_axis_tlast : Inport  Port=4  OutDataTypeStr=boolean  PortDimensions=1  SampleTime=8.33333333333333e-09
  AND : Logic  AllPortsSameDT=off  OutDataTypeStr=boolean  SampleTime=8.33333333333333e-09
  Edge Slice : hdlsllib/Logic and Bit Operations/Bit Slice  lidx=double(8)  ridx=double(8)
      settings: SourceProductName=Simulink  SourceProductBaseCode=SL
  Extract Active Votes : Subsystem
  Gradient Kernel System : Subsystem
  Selector1 : Selector  NumberOfDimensions=2  IndexMode=Zero-based  SampleTime=8.33333333333333e-09  IndexOptions=Index vector (dialog),Index vector (port)  Indices=double(0),double(1)  OutputSizes=double(1),double(1)
  Selector6 : Selector  NumberOfDimensions=2  IndexMode=Zero-based  SampleTime=8.33333333333333e-09  IndexOptions=Index vector (dialog),Index vector (port)  Indices=double(0),double(1)  OutputSizes=double(1),double(1)
  Theta Slice : hdlsllib/Logic and Bit Operations/Bit Slice  lidx=double(7)  ridx=double(0)
      settings: SourceProductName=Simulink  SourceProductBaseCode=SL
  X Counter : hdlsllib/Sources/HDL Counter  CountType=Count limited  CountInit=double(-320)  CountStep=double(1)  CountMax=double(319)  CountFromType=Initial value  CountFrom=double(-320)  CountResetPort=off  CountLoadPort=off  CountEnbPort=on  CountDirPort=off  CountDataType=Signed  CountWordLen=10  CountFracLen=0  CountSampTime=8.33333333333333e-09
      settings: SourceProductName=Simulink
  Y Counter : hdlsllib/Sources/HDL Counter  CountType=Count limited  CountInit=double(-240)  CountStep=double(1)  CountMax=double(239)  CountFromType=Initial value  CountFrom=double(-240)  CountResetPort=off  CountLoadPort=off  CountEnbPort=on  CountDirPort=off  CountDataType=Signed  CountWordLen=9  CountFracLen=0  CountSampTime=8.33333333333333e-09
      settings: SourceProductName=Simulink
  delayMatch : Delay  DelayLength=double(1)  InitialCondition=0  SampleTime=8.33333333333333e-09
  m_axis_tvalid : Outport
  m_axis_tuser : Outport  Port=2
  m_axis_tlast : Outport  Port=3
  hough_param : Outport  Port=4
  edge : Outport  Port=5
  shift : Outport  Port=6
  wires:
  Extract Active Votes/1(Index) -> Selector1/2, delayMatch/1
  s_axis_tlast/1 -> m_axis_tlast/1, AND/2
  s_axis_tuser/1 -> m_axis_tuser/1
  s_axis_tdata/1 -> Edge Slice/1, Theta Slice/1
  s_axis_tvalid/1 -> m_axis_tvalid/1, X Counter/1, AND/1
  Y Counter/1 -> Gradient Kernel System/3(Y)
  X Counter/1 -> Gradient Kernel System/2(X)
  Theta Slice/1 -> Extract Active Votes/1(Theta), Gradient Kernel System/4(Theta)
  Selector6/1 -> hough_param/1
  Selector1/1 -> shift/1
  Gradient Kernel System/3(Shift) -> Selector1/1
  Gradient Kernel System/2(Rho) -> Selector6/1
  Gradient Kernel System/1(vEdge) -> edge/1
  delayMatch/1 -> Selector6/2
  Edge Slice/1 -> Gradient Kernel System/1(Edge)
  AND/1 -> Y Counter/1

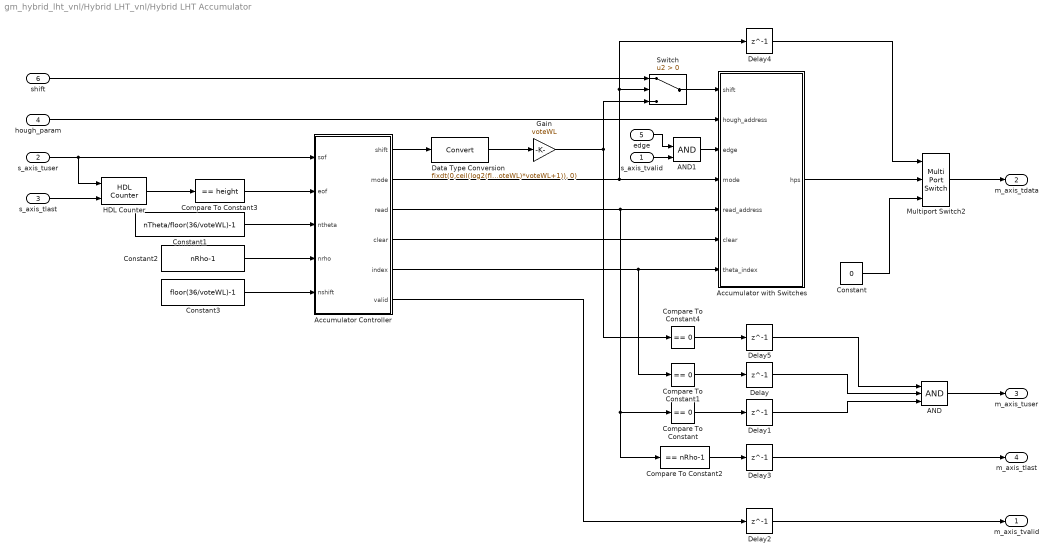
== system gm_hybrid_lht_vnl/Hybrid LHT_vnl/Hybrid LHT Accumulator ==
  s_axis_tvalid : Inport
  s_axis_tuser : Inport  Port=2
  s_axis_tlast : Inport  Port=3
  hough_param : Inport  Port=4
  edge : Inport  Port=5
  shift : Inport  Port=6
  AND : Logic  Inputs=3  IconShape=distinctive  AllPortsSameDT=off  OutDataTypeStr=boolean
  AND1 : Logic  IconShape=distinctive  AllPortsSameDT=off  OutDataTypeStr=boolean
  Accumulator Controller : MATLAB Function  TreatAsAtomicUnit=on
  Accumulator with Switches : Subsystem
  Compare To Constant : simulink/Logic and Bit Operations/Compare To Constant  relop===  const=0  OutDataTypeStr=boolean
  Compare To Constant1 : simulink/Logic and Bit Operations/Compare To Constant  relop===  const=0  OutDataTypeStr=boolean
  Compare To Constant2 : simulink/Logic and Bit Operations/Compare To Constant  relop===  const=nRho-1  OutDataTypeStr=boolean
  Compare To Constant3 : simulink/Logic and Bit Operations/Compare To Constant  relop===  const=height  OutDataTypeStr=boolean
  Compare To Constant4 : simulink/Logic and Bit Operations/Compare To Constant  relop===  const=0  OutDataTypeStr=boolean
  Constant : Constant  Value=0  OutDataTypeStr=fixdt(0, ceil(log2(2*maxRho)), 0)  SampleTime=-1
  Constant1 : Constant  Value=nTheta/floor(36/voteWL)-1  OutDataTypeStr=uint16  SampleTime=-1
  Constant2 : Constant  Value=nRho-1  OutDataTypeStr=uint16  SampleTime=-1
  Constant3 : Constant  Value=floor(36/voteWL)-1  OutDataTypeStr=fixdt(0, floor(36/voteWL), 0)  SampleTime=-1
  Data Type Conversion : DataTypeConversion  OutDataTypeStr=fixdt(0,ceil(log2(floor(36/voteWL)*voteWL+1)), 0)
  Delay{,1..5} (6 alike) : Delay  DelayLength=1
  Gain : Gain  Gain=voteWL  OutDataTypeStr=fixdt(0,ceil(log2(floor(36/voteWL)*voteWL+1)), 0)
  HDL Counter : hdlsllib/Sources/HDL Counter  CountType=Count limited  CountInit=0  CountStep=1  CountMax=height  CountFromType=Initial value  CountFrom=0  CountResetPort=on  CountLoadPort=off  CountEnbPort=on  CountDirPort=off  CountDataType=Unsigned  CountWordLen=ceil(log2(height+1))  CountFracLen=0  CountSampTime=1
      settings: SourceProductName=Simulink
  Multiport Switch2 : MultiPortSwitch  DataPortOrder=Zero-based contiguous  Inputs=2  zeroidx=on
  Switch : Switch  Criteria=u2 > Threshold
  m_axis_tvalid : Outport
  m_axis_tdata : Outport  Port=2
  m_axis_tuser : Outport  Port=3
  m_axis_tlast : Outport  Port=4
  wires:
  s_axis_tvalid/1 -> AND1/2
  AND1/1 -> Accumulator with Switches/3(edge)
  edge/1 -> AND1/1
  Data Type Conversion/1 -> Gain/1
  Gain/1 -> Compare To Constant4/1, Switch/3
  Constant3/1 -> Accumulator Controller/5(nshift)
  Delay/1 -> AND/2
  Delay1/1 -> AND/3
  Compare To Constant4/1 -> Delay5/1
  Delay5/1 -> AND/1
  Accumulator Controller/1(shift) -> Data Type Conversion/1
  shift/1 -> Switch/1
  Switch/1 -> Accumulator with Switches/1(shift)
  Accumulator Controller/4(clear) -> Accumulator with Switches/6(clear)
  Accumulator Controller/2(mode) -> Delay4/1, Switch/2, Accumulator with Switches/4(mode)
  Accumulator Controller/3(read) -> Accumulator with Switches/5(read_address), Compare To Constant2/1, Compare To Constant/1
  Constant1/1 -> Accumulator Controller/3(ntheta)
  Accumulator Controller/5(index) -> Compare To Constant1/1, Accumulator with Switches/7(theta_index)
  Compare To Constant2/1 -> Delay3/1
  Constant2/1 -> Accumulator Controller/4(nrho)
  s_axis_tuser/1 -> Accumulator Controller/1(sof), HDL Counter/1
  Compare To Constant1/1 -> Delay/1
  Compare To Constant/1 -> Delay1/1
  Delay3/1 -> m_axis_tlast/1
  hough_param/1 -> Accumulator with Switches/2(hough_address)
  AND/1 -> m_axis_tuser/1
  HDL Counter/1 -> Compare To Constant3/1
  s_axis_tlast/1 -> HDL Counter/2
  Compare To Constant3/1 -> Accumulator Controller/2(eof)
  Multiport Switch2/1 -> m_axis_tdata/1
  Accumulator with Switches/1(hps) -> Multiport Switch2/2
  Constant/1 -> Multiport Switch2/3
  Accumulator Controller/6(valid) -> Delay2/1
  Delay2/1 -> m_axis_tvalid/1
  Delay4/1 -> Multiport Switch2/1

== system gm_hybrid_lht_vnl/Hybrid LHT_vnl/Hybrid LHT Kernel ==
  s_axis_tvalid : Inport
  s_axis_tdata : Inport  Port=2
  s_axis_tuser : Inport  Port=3
  s_axis_tlast : Inport  Port=4
  AND : Logic  IconShape=distinctive  AllPortsSameDT=off  OutDataTypeStr=boolean
  Edge Slice : hdlsllib/Logic and Bit Operations/Bit Slice  lidx=ceil(log2(round(theta(end)/dTheta)+1))  ridx=ceil(log2(round(theta(end)/dTheta)+1))
      settings: SourceProductName=Simulink  SourceProductBaseCode=SL
  Extract Active Votes : Subsystem
  Gradient Kernel System : Subsystem
  Selector1 : Selector  NumberOfDimensions=2  IndexMode=Zero-based  InputPortWidth=3  IndexOptions=Index vector (dialog),Index vector (port)  Indices=0,1  OutputSizes=1,1
  Selector6 : Selector  NumberOfDimensions=2  IndexMode=Zero-based  InputPortWidth=3  IndexOptions=Index vector (dialog),Index vector (port)  Indices=0,1  OutputSizes=1,1
  Theta Slice : hdlsllib/Logic and Bit Operations/Bit Slice  lidx=ceil(log2(round(theta(end)/dTheta)+1))-1  ridx=0
      settings: SourceProductName=Simulink  SourceProductBaseCode=SL
  X Counter : hdlsllib/Sources/HDL Counter  CountType=Count limited  CountInit=-width/2  CountStep=1  CountMax=width/2-1  CountFromType=Initial value  CountFrom=-width/2  CountResetPort=off  CountLoadPort=off  CountEnbPort=on  CountDirPort=off  CountDataType=Signed  CountWordLen=ceil(log2(width))  CountFracLen=0  CountSampTime=1
      settings: SourceProductName=Simulink
  Y Counter : hdlsllib/Sources/HDL Counter  CountType=Count limited  CountInit=-height/2  CountStep=1  CountMax=height/2-1  CountFromType=Initial value  CountFrom=-height/2  CountResetPort=off  CountLoadPort=off  CountEnbPort=on  CountDirPort=off  CountDataType=Signed  CountWordLen=ceil(log2(height))  CountFracLen=0  CountSampTime=1
      settings: SourceProductName=Simulink
  m_axis_tvalid : Outport
  m_axis_tuser : Outport  Port=2
  m_axis_tlast : Outport  Port=3
  hough_param : Outport  Port=4
  edge : Outport  Port=5
  shift : Outport  Port=6
  wires:
  Y Counter/1 -> Gradient Kernel System/3(Y)
  X Counter/1 -> Gradient Kernel System/2(X)
  s_axis_tdata/1 -> Theta Slice/1, Edge Slice/1
  AND/1 -> Y Counter/1
  Gradient Kernel System/1(vEdge) -> edge/1
  Gradient Kernel System/3(Shift) -> Selector1/1
  Gradient Kernel System/2(Rho) -> Selector6/1
  Extract Active Votes/1(Index) -> Selector1/2, Selector6/2
  Selector6/1 -> hough_param/1
  Selector1/1 -> shift/1
  Edge Slice/1 -> Gradient Kernel System/1(Edge)
  Theta Slice/1 -> Extract Active Votes/1(Theta), Gradient Kernel System/4(Theta)
  s_axis_tuser/1 -> m_axis_tuser/1
  s_axis_tlast/1 -> m_axis_tlast/1, AND/2
  s_axis_tvalid/1 -> m_axis_tvalid/1, X Counter/1, AND/1

== system gm_hybrid_lht_vnl/Hybrid LHT/Hybrid LHT Accumulator/Accumulator Controller ==
  sof : Inport  OutDataTypeStr=boolean  PortDimensions=1  SampleTime=8.33333333333333e-09
  eof : Inport  Port=2  OutDataTypeStr=boolean  PortDimensions=1  SampleTime=8.33333333333333e-09
  ntheta : Inport  Port=3  OutDataTypeStr=uint16  PortDimensions=1  SampleTime=8.33333333333333e-09
  nrho : Inport  Port=4  OutDataTypeStr=uint16  PortDimensions=1  SampleTime=8.33333333333333e-09
  nshift : Inport  Port=5  OutDataTypeStr=fixdt(0, 3, 0)  PortDimensions=1  SampleTime=8.33333333333333e-09
  Accumulator Controller : MATLAB Function  TreatAsAtomicUnit=on
  shift : Outport
  mode : Outport  Port=2
  read : Outport  Port=3
  clear : Outport  Port=4
  index : Outport  Port=5
  valid : Outport  Port=6
  wires:
  nshift/1 -> Accumulator Controller/5(nshift)
  nrho/1 -> Accumulator Controller/4(nrho)
  ntheta/1 -> Accumulator Controller/3(ntheta)
  eof/1 -> Accumulator Controller/2(eof)
  sof/1 -> Accumulator Controller/1(sof)
  Accumulator Controller/6(valid) -> valid/1
  Accumulator Controller/5(index) -> index/1
  Accumulator Controller/4(clear) -> clear/1
  Accumulator Controller/3(read) -> read/1
  Accumulator Controller/2(mode) -> mode/1
  Accumulator Controller/1(shift) -> shift/1
